simulink model "pend_m_motor"  (R2022a)
settings: Solver=FixedStepAuto  StartTime=0.0  StopTime=SIM_TIME  FixedStep=STEP_SIZE  RelTol=1e-3
undefined symbols (not defined in the file): a_st, B, b, c, dtheta0, dx0, FN, g, I, Jd, ke, kt, l, M, m, mu_k, mu_s, mu_v, r, R, theta0, x0
settings Model: Creator=farfar  LastModifiedBy=farfar
settings DataIOCC: ReturnWorkspaceOutputs=off

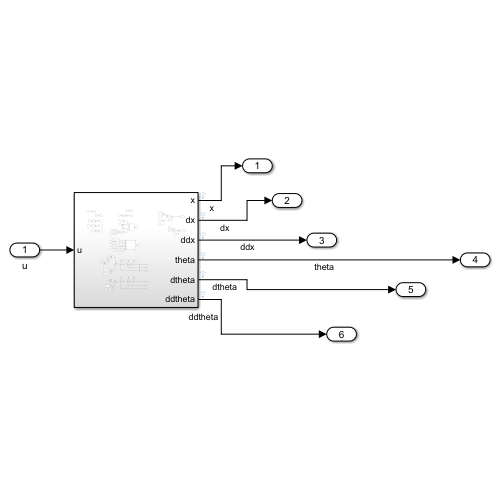
[thumbnail: Simulink's stored preview of the top-level diagram]
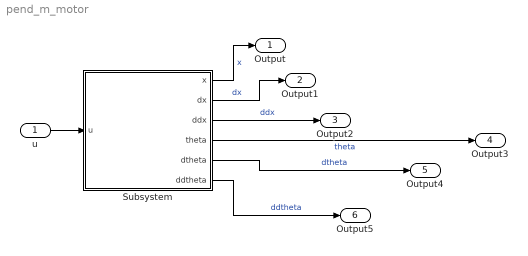
== system pend_m_motor ==
  u : Inport
  Subsystem : Subsystem
  Output : Outport
  Output1 : Outport  Port=2
  Output2 : Outport  Port=3
  Output3 : Outport  Port=4
  Output4 : Outport  Port=5
  Output5 : Outport  Port=6
  wires:
  u/1 -> Subsystem/1(u)
  Subsystem/1(x) -> Output/1  "x"
  Subsystem/2(dx) -> Output1/1  "dx"
  Subsystem/3(ddx) -> Output2/1  "ddx"
  Subsystem/4(theta) -> Output3/1  "theta"
  Subsystem/5(dtheta) -> Output4/1  "dtheta"
  Subsystem/6(ddtheta) -> Output5/1  "ddtheta"

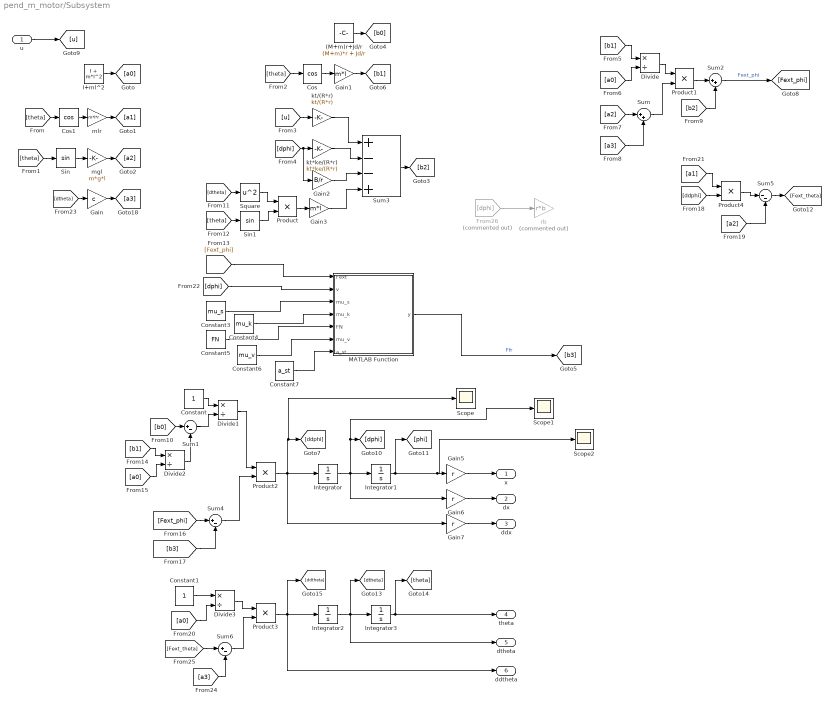
== system pend_m_motor/Subsystem ==
  u : Inport
  (M+m)r+Jd/r : Constant  Value=(M+m)*r + Jd/r
  Constant : Constant
  Constant1 : Constant
  Constant3 : Constant  Value=mu_s
  Constant4 : Constant  Value=mu_k
  Constant5 : Constant  Value=FN
  Constant6 : Constant  Value=mu_v
  Constant7 : Constant  Value=a_st
  Cos : Trigonometry  Operator=cos
  Cos1 : Trigonometry  Operator=cos
  Divide{,1..3} (4 alike) : Product  Inputs=*/
  From26 : From  Commented=on  GotoTag=dphi
  Gain : Gain  Gain=c
  Gain1 : Gain  Gain=m*l
  Gain2 : Gain  Gain=B/r
  Gain3 : Gain  Gain=m*l
  Gain5 : Gain  Gain=r
  Gain6 : Gain  Gain=r
  Gain7 : Gain  Gain=r
  I+ml^2 : Constant  Value=I + m*l^2
  Integrator : Integrator  InitialCondition=dx0/r
  Integrator1 : Integrator  InitialCondition=x0/r
  Integrator2 : Integrator  InitialCondition=dtheta0
  Integrator3 : Integrator  InitialCondition=theta0
  MATLAB Function : MATLAB Function  TreatAsAtomicUnit=on
  Product{,1..4} (5 alike) : Product
  Scope : Scope
  Scope1 : Scope
  Scope2 : Scope
  Sin : Trigonometry
  Sin1 : Trigonometry
  Square : Math  Operator=square
  Sum : Sum  Inputs=|++
  Sum1 : Sum  Inputs=|+-
  Sum2 : Sum  Inputs=|++
  Sum3 : Sum  Inputs=+--+
  Sum4 : Sum  Inputs=|+-
  Sum5 : Sum  Inputs=|--
  Sum6 : Sum  Inputs=|+-
  kt*ke/(R*r) : Gain  Gain=kt*ke/(R*r)
  kt/(R*r) : Gain  Gain=kt/(R*r)
  mgl : Gain  Gain=m*g*l
  mlr : Gain  Gain=m*l*r
  rb : Gain  Commented=on  Gain=r*b
  x : Outport
  dx : Outport  Port=2
  ddx : Outport  Port=3
  theta : Outport  Port=4
  dtheta : Outport  Port=5
  ddtheta : Outport  Port=6
  wires:
  (M+m)r+Jd/r/1 -> [b0]
  I+ml^2/1 -> [a0]
  [theta] -> Sin/1
  u/1 -> [u]
  Sum2/1 -> [Fext_phi]  "Fext_phi"
  Constant4/1 -> MATLAB Function/4(mu_k)
  Sin/1 -> mgl/1
  Constant7/1 -> MATLAB Function/7(a_st)
  [Fext_phi] -> MATLAB Function/1(Fext)
  Constant3/1 -> MATLAB Function/3(mu_s)
  Constant5/1 -> MATLAB Function/5(FN)
  Cos1/1 -> mlr/1
  [theta] -> Cos1/1
  mlr/1 -> [a1]
  mgl/1 -> [a2]
  Gain/1 -> [a3]
  [dtheta] -> Gain/1
  Gain1/1 -> [b1]
  Cos/1 -> Gain1/1
  [theta] -> Cos/1
  [u] -> kt/(R*r)/1
  [dphi] -> Gain2/1, kt*ke/(R*r)/1
  kt/(R*r)/1 -> Sum3/1
  kt*ke/(R*r)/1 -> Sum3/2
  Gain2/1 -> Sum3/3
  Sum3/1 -> [b2]
  Product/1 -> Gain3/1
  Square/1 -> Product/1
  [dtheta] -> Square/1
  Sin1/1 -> Product/2
  [theta] -> Sin1/1
  Gain3/1 -> Sum3/4
  [dphi] -> MATLAB Function/2(v)
  [b1] -> Divide/1
  [a0] -> Divide/2
  Divide/1 -> Product1/1
  [a2] -> Sum/1
  [a3] -> Sum/2
  Sum/1 -> Product1/2
  [b2] -> Sum2/2
  Product1/1 -> Sum2/1
  Constant6/1 -> MATLAB Function/6(mu_v)
  Constant/1 -> Divide1/1
  [b0] -> Sum1/1
  Divide2/1 -> Sum1/2
  [a0] -> Divide2/2
  [b1] -> Divide2/1
  Sum1/1 -> Divide1/2
  Product2/1 -> Gain7/1, Integrator/1, Scope/1, [ddphi]
  Divide1/1 -> Product2/1
  Sum4/1 -> Product2/2
  [Fext_phi] -> Sum4/1
  [b3] -> Sum4/2
  Integrator/1 -> Gain6/1, Scope1/1, [dphi], Integrator1/1
  Integrator1/1 -> Scope2/1, Gain5/1, [phi]
  [a2] -> Sum5/2
  Sum5/1 -> [Fext_theta]
  Divide3/1 -> Product3/1
  Constant1/1 -> Divide3/1
  [ddphi] -> Product4/2
  Product4/1 -> Sum5/1
  [a1] -> Product4/1
  [a0] -> Divide3/2
  Sum6/1 -> Product3/2
  [a3] -> Sum6/2
  [Fext_theta] -> Sum6/1
  Integrator3/1 -> theta/1, [theta]
  Integrator2/1 -> dtheta/1, [dtheta], Integrator3/1
  Product3/1 -> ddtheta/1, Integrator2/1, [ddtheta]
  Gain5/1 -> x/1
  Gain6/1 -> dx/1
  Gain7/1 -> ddx/1
  From26/1 -> rb/1
  MATLAB Function/1(y) -> [b3]  "Ffr"

== matlab function pend_m_motor/Subsystem/MATLAB Function ==
  data: Fext input; y output; v input; mu_s input; mu_k input; FN input; mu_v input; a_st input
function y = fcn(Fext, v, mu_s, mu_k, FN, mu_v, a_st)
%mu_s = 1.5;
%mu_k = 0.5;
%mu_v = 0.3;
%a_st = 1;
%FN = 10*9.8;
Fs = mu_s * FN;% * sign(v);
Fk = mu_k * FN;% * sign(v);
Fv = 0;%mu_v * FN;

v_tol = 0.00000000000000001;
y = 0;
opt = 0;
if and(abs(v) <= v_tol, Fext < Fs)
    y = Fext;
    opt = 1;
elseif and(abs(v) <= v_tol, Fext >= Fs)
    y = Fs;
    opt = 2;
elseif and(abs(v) > v_tol, v > 0)
    y = Fk + (Fs - Fk)*exp(-a_st * v) + Fv * v;
    opt = 3;
elseif and(abs(v) > v_tol, v < 0) 
    y = -Fk + (Fk - Fs)*exp(a_st * v) - Fv * v;
    opt = 4;
end
